simulink model "problem_3"  (R2020b)
settings: Solver=VariableStepAuto  StartTime=0.0  StopTime=10.0  RelTol=1e-3
settings Model: Creator=k.Raviteja  LastModifiedBy=k.Raviteja

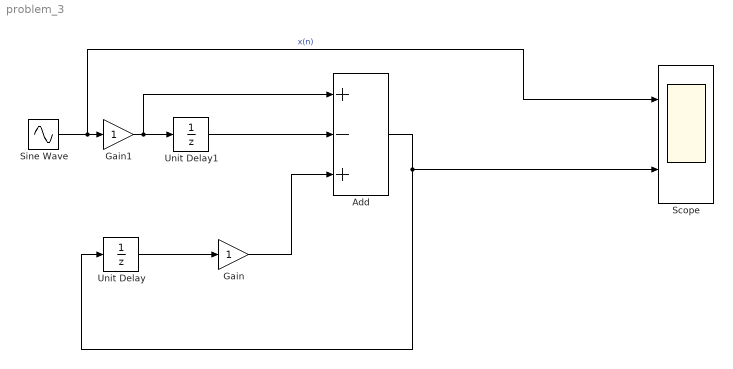
== system problem_3 ==
  Add : Sum  Inputs=+-+
  Gain : Gain
  Gain1 : Gain
  Scope : Scope  NumInputPorts=2
  Sine Wave : Sin  SampleTime=0
  Unit Delay : UnitDelay  SampleTime=-1  HasFrameUpgradeWarning=on
  Unit Delay1 : UnitDelay  SampleTime=-1  HasFrameUpgradeWarning=on
  wires:
  Sine Wave/1 -> Scope/1, Gain1/1  "x(n)"
  Gain1/1 -> Add/1, Unit Delay1/1
  Unit Delay1/1 -> Add/2
  Add/1 -> Scope/2, Unit Delay/1
  Unit Delay/1 -> Gain/1
  Gain/1 -> Add/3
